simulink model "FlightSoftware"  (Simulink 7.5)
settings: Solver=ode3  StartTime=0.0  StopTime=10.0  RelTol=1e-3
settings Model: Creator=rruff  LastModifiedBy=rruff
settings OptimizationCC: InlineParams=on
settings RTWCC: ProcessScript=grt_make_rtw_hook

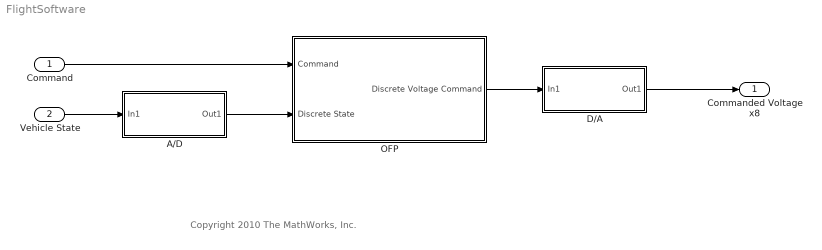
== system FlightSoftware ==
  note: Copyright 2010 The MathWorks, Inc.
  Command : Inport  OutDataType=fixdt(1, 16)  OutScaling=2^0
  Vehicle State : Inport  Port=2  OutDataType=fixdt(1, 16)  OutScaling=2^0
  A/D : Subsystem  TreatAsAtomicUnit=on
  D/A : Subsystem  TreatAsAtomicUnit=on
  OFP : Subsystem  TreatAsAtomicUnit=on
  Commanded Voltage x8 : Outport  OutDataType=fixdt(1, 16)  OutScaling=2^0
  wires:
  OFP/1(Discrete Voltage Command) -> D/A/1(In1)
  Vehicle State/1 -> A/D/1(In1)
  A/D/1(Out1) -> OFP/2(Discrete State)
  D/A/1(Out1) -> Commanded Voltage x8/1
  Command/1 -> OFP/1(Command)

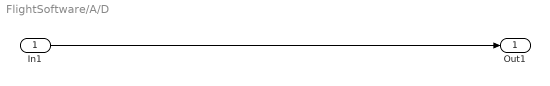
== system FlightSoftware/A/D ==
  In1 : Inport  OutDataType=fixdt(1, 16)  OutScaling=2^0
  Out1 : Outport  OutDataType=fixdt(1, 16)  OutScaling=2^0
  wires:
  In1/1 -> Out1/1

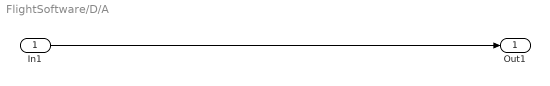
== system FlightSoftware/D/A ==
  In1 : Inport  OutDataType=fixdt(1, 16)  OutScaling=2^0
  Out1 : Outport  OutDataType=fixdt(1, 16)  OutScaling=2^0
  wires:
  In1/1 -> Out1/1

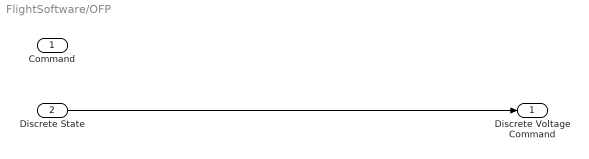
== system FlightSoftware/OFP ==
  Command : Inport  PortDimensions=1  SampleTime=0.01  OutMin=0  OutMax=10  DataType=double  OutDataType=fixdt(1, 16)  OutScaling=2^0  OutDataTypeStr=double
  Discrete State : Inport  Port=2  PortDimensions=12  SampleTime=0.01  DataType=double  OutDataType=fixdt(1, 16)  OutScaling=2^0  OutDataTypeStr=double
  Discrete Voltage Command : Outport  PortDimensions=8  SampleTime=0.01  OutMin=0  OutMax=5  DataType=double  OutDataType=fixdt(1, 16)  OutScaling=2^0  OutDataTypeStr=double
  wires:
  Discrete State/1 -> Discrete Voltage Command/1
